simulink model "example_Storage_Type11"  (R2018b)
settings: Solver=ode45  StartTime=0.0  StopTime=7000  MaxStep=300  RelTol=1e-3  EnableMultiTasking=on
undefined symbols (not defined in the file): path_carnot
libraries: carnot x11, simulink x4
settings Model: Creator=drhf  LastModifiedBy=P41573
settings DataIOCC: LimitDataPoints=on  SaveFormat=Array
settings OptimizationCC: ExpressionDepthLimit=2147483647  LifeSpan=inf
settings DebuggingCC: UnderspecifiedInitializationDetection=Classic  MergeDetectMultiDrivingBlocksExec=none  SolverPrmCheckMsg=warning  StateNameClashWarn=warning  SFUnexpectedBacktrackingDiag=warning  SFNoUnconditionalDefaultTransitionDiag=warning  SFExecutionAtInitializationDiag=none
settings HardwareCC: ProdBitPerPointer=32  ProdBitPerSizeT=32  ProdBitPerPtrDiffT=32  ProdLargestAtomicFloat=None  ProdIntDivRoundTo=Undefined  ProdEndianess=Unspecified  ProdWordSize=32  ProdHWDeviceType=32-bit Generic
settings ModelReferenceCC: PropagateSignalLabelsOutOfModel=off
settings SFSimCC: SimUseLocalCustomCode=off
settings RTWCC: RTWUseLocalCustomCode=off
settings CodeAppCC: StateflowObjectComments=on
settings GRTTargetCC: TargetLangStandard=C89/C90 (ANSI)  GeneratePreprocessorConditionals=Disable all  CombineOutputUpdateFcns=off  GRTInterface=on
settings ConfigComp: CovMetricSettings=dw  CovHtmlReporting=on  CovSaveCumulativeToWorkspaceVar=on  CovSaveSingleToWorkspaceVar=on  CovExternalEMLEnable=off

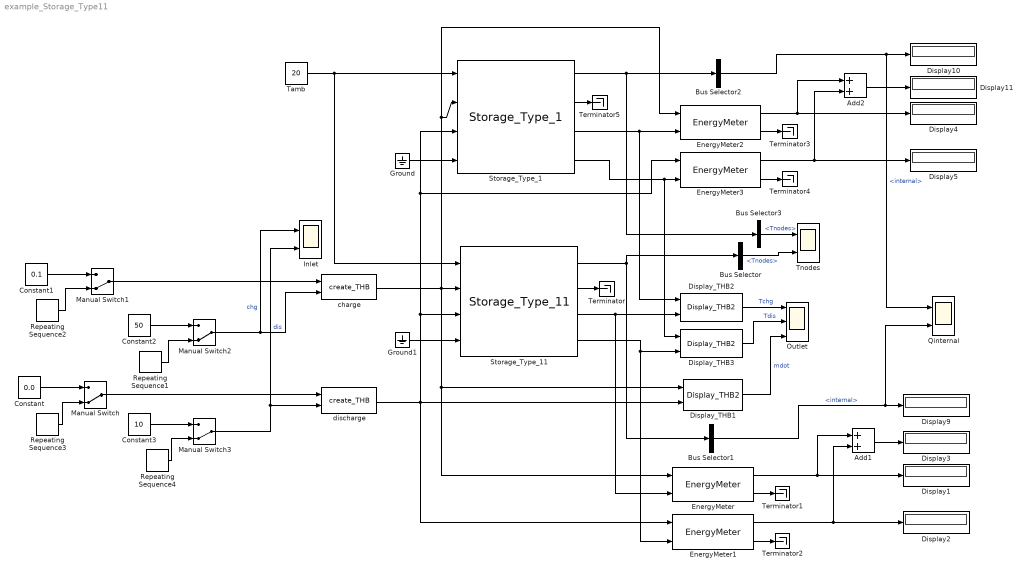
== system example_Storage_Type11 ==
  Add1 : Sum  Inputs=2
  Add2 : Sum  Inputs=2
  Bus Selector : BusSelector  OutputSignals=Tnodes
  Bus Selector1 : BusSelector  OutputSignals=energy.internal
  Bus Selector2 : BusSelector  OutputSignals=energy.internal
  Bus Selector3 : BusSelector  OutputSignals=Tnodes
  Constant : Constant  Value=0.0
  Constant1 : Constant  Value=0.1
  Constant2 : Constant  Value=50
  Constant3 : Constant  Value=10
  Display{1..5,9..11} (8 alike) : Display
  Display_THB1 : carnot/Outputs/Display_THB2  t=off  m=on  p=off  id=off  mix=off  d=off
      settings: SourceProductName=Carnot
  Display_THB2 : carnot/Outputs/Display_THB2  t=on  m=off  p=off  id=off  mix=off  d=off
      settings: SourceProductName=Carnot
  Display_THB3 : carnot/Outputs/Display_THB2  t=on  m=off  p=off  id=off  mix=off  d=off
      settings: SourceProductName=Carnot
  EnergyMeter{,1..3} (4 alike) : carnot/Control/EnergyMeter
      settings: SourceProductName=Carnot
  Ground : Ground
  Ground1 : Ground
  Inlet : Scope  NumInputPorts=2
  Manual Switch{,1..3} (4 alike) : ManualSwitch  CurrentSetting=0
  Outlet : Scope  NumInputPorts=3
  Qinternal : Scope  NumInputPorts=2
  Repeating Sequence1 : simulink/Sources/Repeating Sequence  rep_seq_t=[0 1000 1200 1400 7000]  rep_seq_y=[50 50 20 50 50]
  Repeating Sequence2 : simulink/Sources/Repeating Sequence  rep_seq_t=[0 3600 3700 6400 6500 7000]  rep_seq_y=[0.4 0.4 0.1 0.1 0 0]
  Repeating Sequence3 : simulink/Sources/Repeating Sequence  rep_seq_t=[0 3500 3600 7000]  rep_seq_y=[0.1 0.1 0.4 0.4]
  Repeating Sequence4 : simulink/Sources/Repeating Sequence  rep_seq_t=[0 3700 3800 3900 7000]  rep_seq_y=[10 10 40 10 10]
  Storage_Type_1 : carnot/Storage/Thermal/Storage_Type_1  t0=10  hgt=1.7684  stgtype=1  tini=[10 10 10 10 10 10 10 10 10 10]  mpts=[1 2 3 4 5 6 7 8 9 10]  PathName=fullfile(path_carnot('libsl'),'Storage','Thermal','Storage_Type_1','parameter_set')  FileName='<user defined>'  userPath=off  userParam=on  uwall=1  ubot=1  utop=1  axcond=1  volume=0.5  dia=0.6  standing=standing cylinder  nodes=10  mpoints=10  Tsensor=0.5  pipe1inlet=1  pipe1outlet=0  pipe1dia=0.03  pipe2inlet=0.1  pipe2outlet=1  pipe2dia=0.03  heater1start=0.6  heater1end=0.65
      settings: SourceProductName=Carnot
  Storage_Type_11 : carnot/Storage/Thermal/Storage_Type_11  t0=10  hgt=1.7684  stgtype=11  tini=[10 10 10 10 10 10 10 10 10 10]  mpts=[1 2 3 4 5 6 7 8 9 10]  PathName=fullfile(path_carnot('libsl'), 'Storage', 'Thermal', 'Storage_Type_11', 'parameter_set')  FileName='StorageType11_500_L.mat'  userPath=off  userParam=off  uwall=1  ubot=1  utop=1  axcond=1  volume=0.5  dia=0.6  standing=standing cylinder  nodes=10  mpoints=10  Tsensor=0.5  vTpiece=0.004  pipe1inlet=1  pipe1outlet=0  pipe1dia=0.03  pipe2inlet=0.1  pipe2outlet=1  pipe2dia=0.03  heater1start=0.6  heater1end=0.65
      settings: SourceProductName=Carnot
  Tamb : Constant  Value=20
  Terminator{,1..5} (6 alike) : Terminator
  Tnodes : Scope  NumInputPorts=2
  charge : carnot/Source/Simple/create_THB  p=1e5  fluid=Water  mix=0  mix2=0  mix3=0  dia=0  hgt=0  mID=No Pressure Drop
      settings: SourceProductName=Carnot
  discharge : carnot/Source/Simple/create_THB  p=1e5  fluid=Water  mix=0  mix2=0  mix3=0  dia=0  hgt=0  mID=No Pressure Drop
      settings: SourceProductName=Carnot
  wires:
  Tamb/1 -> Storage_Type_11/1, Storage_Type_1/1
  charge/1 -> Storage_Type_11/2, EnergyMeter/1, Display_THB1/1, Storage_Type_1/2, EnergyMeter2/1
  discharge/1 -> EnergyMeter1/1, Display_THB1/2, Storage_Type_1/3, EnergyMeter3/1, Storage_Type_11/3
  Storage_Type_11/3 -> Display_THB2/2, EnergyMeter/2
  Storage_Type_11/4 -> Display_THB3/2, EnergyMeter1/2
  Display_THB2/1 -> Outlet/1  "Tchg"
  Display_THB1/1 -> Outlet/3  "mdot"
  Storage_Type_11/2 -> Terminator/1
  Storage_Type_11/1 -> Bus Selector1/1, Bus Selector/1
  Bus Selector/1 -> Tnodes/2  "<Tnodes>"
  Bus Selector1/1 -> Qinternal/2, Display9/1  "<internal>"
  EnergyMeter/2 -> Terminator1/1
  EnergyMeter/1 -> Add1/1, Display1/1
  EnergyMeter1/1 -> Add1/2, Display2/1
  EnergyMeter1/2 -> Terminator2/1
  Storage_Type_1/1 -> Bus Selector3/1, Bus Selector2/1
  Storage_Type_1/2 -> Terminator5/1
  Storage_Type_1/3 -> Display_THB2/1, EnergyMeter2/2
  Storage_Type_1/4 -> Display_THB3/1, EnergyMeter3/2
  Bus Selector3/1 -> Tnodes/1  "<Tnodes>"
  Bus Selector2/1 -> Qinternal/1, Display10/1  "<internal>"
  EnergyMeter3/1 -> Add2/2, Display5/1
  EnergyMeter3/2 -> Terminator4/1
  EnergyMeter2/1 -> Add2/1, Display4/1
  EnergyMeter2/2 -> Terminator3/1
  Add1/1 -> Display3/1
  Add2/1 -> Display11/1
  Manual Switch1/1 -> charge/1
  Manual Switch/1 -> discharge/1
  Manual Switch2/1 -> Inlet/1, charge/2  "chg"
  Manual Switch3/1 -> Inlet/2, discharge/2  "dis"
  Display_THB3/1 -> Outlet/2  "Tdis"
  Repeating Sequence3/1 -> Manual Switch/2
  Repeating Sequence2/1 -> Manual Switch1/2
  Constant/1 -> Manual Switch/1
  Constant1/1 -> Manual Switch1/1
  Constant2/1 -> Manual Switch2/1
  Repeating Sequence1/1 -> Manual Switch2/2
  Constant3/1 -> Manual Switch3/1
  Repeating Sequence4/1 -> Manual Switch3/2
  Ground/1 -> Storage_Type_1/4
  Ground1/1 -> Storage_Type_11/4
